simulink model "eulerEq"  (R2023b)
settings: Solver=ode4  StartTime=0.0  StopTime=30000  FixedStep=0.01  RelTol=1e-3
values from neighbouring files (symbols this model uses):
  date = [2023, 1, 21, 13, 52, 0]    [main.m]    (also in main_nonLin.m)
  euler0 = [0; 0; 0]    [main.m]    (also in main_nonLin.m)
  w0 = h0./sat.I'    [main.m]    (also in main_nonLin.m)
undefined symbols (not defined in the file or in its folder): airDensity, astroConstants, control, DiscIntNeverNeededParam, ea0, earth, gyroscope, magneticConstants, magnetorquer, magSensor, orbit, physicsConstants, rw, sat, sunSensor
libraries: simulink x21, matrix_library x7, sharedtransform x5, dspindex x5, sharedutil x4, vrlib x3, dspfactors x1, simulink_extras x1
(part 2 of 2)

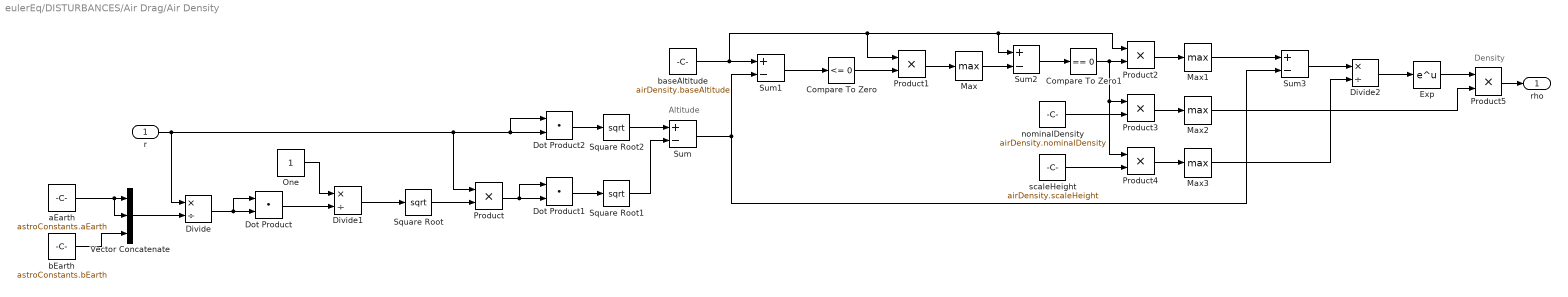
== system eulerEq/DISTURBANCES/Air Drag/Air Density ==
  note: Density
  note: Altitude
  r : Inport
  Compare To Zero : simulink/Logic and Bit Operations/Compare To Zero  relop=<=  OutDataTypeStr=boolean
  Compare To Zero1 : simulink/Logic and Bit Operations/Compare To Zero  relop===  OutDataTypeStr=boolean
  Divide : Product  Inputs=*/
  Divide1 : Product  Inputs=*/
  Divide2 : Product  Inputs=*/
  Dot Product : DotProduct  OutDataTypeStr=Inherit: Inherit via internal rule
  Dot Product1 : DotProduct  OutDataTypeStr=Inherit: Inherit via internal rule
  Dot Product2 : DotProduct  OutDataTypeStr=Inherit: Inherit via internal rule
  Exp : Math
  Max{,1..3} (4 alike) : MinMax  Function=max
  One : Constant  OutDataTypeStr=Inherit: Inherit via back propagation
  Product{,1..5} (6 alike) : Product
  Square Root : Sqrt
  Square Root1 : Sqrt
  Square Root2 : Sqrt
  Sum{,1..3} (4 alike) : Sum  Inputs=+-
  Vector Concatenate : Concatenate  NumInputs=3
  aEarth : Constant  Value=astroConstants.aEarth
  bEarth : Constant  Value=astroConstants.bEarth
  baseAltitude : Constant  Value=airDensity.baseAltitude
  nominalDensity : Constant  Value=airDensity.nominalDensity
  scaleHeight : Constant  Value=airDensity.scaleHeight
  rho : Outport
  wires:
  Product4/1 -> Max3/1
  Product/1 -> Dot Product1/1, Dot Product1/2
  Sum/1 -> Sum1/2, Sum3/2
  Max2/1 -> Product5/2
  Dot Product1/1 -> Square Root1/1
  Divide2/1 -> Exp/1
  Exp/1 -> Product5/1
  aEarth/1 -> Vector Concatenate/2, Vector Concatenate/1
  Product3/1 -> Max2/1
  Divide/1 -> Dot Product/1, Dot Product/2
  baseAltitude/1 -> Sum1/1, Product1/1, Sum2/1, Product2/1
  Max1/1 -> Sum3/1
  Dot Product/1 -> Divide1/2
  Max3/1 -> Divide2/2
  Compare To Zero1/1 -> Product2/2, Product4/1, Product3/1
  scaleHeight/1 -> Product4/2
  Dot Product2/1 -> Square Root2/1
  nominalDensity/1 -> Product3/2
  Sum1/1 -> Compare To Zero/1
  Square Root1/1 -> Sum/2
  Sum2/1 -> Compare To Zero1/1
  Sum3/1 -> Divide2/1
  Compare To Zero/1 -> Product1/2
  Product1/1 -> Max/1
  Product5/1 -> rho/1
  Max/1 -> Sum2/2
  bEarth/1 -> Vector Concatenate/3
  One/1 -> Divide1/1
  Divide1/1 -> Square Root/1
  Vector Concatenate/1 -> Divide/2
  Square Root2/1 -> Sum/1
  Square Root/1 -> Product/2
  Product2/1 -> Max1/1
  r/1 -> Divide/1, Dot Product2/1, Dot Product2/2, Product/1

== system eulerEq/DISTURBANCES/Air Drag/Matrix Cross Product ==
  a : Inport
  b : Inport  Port=2
  Add3 : Sum  Inputs=+-
  Add4 : Sum  Inputs=+-
  Add5 : Sum  Inputs=+-
  Matrix Concatenate2 : Concatenate  NumInputs=3  Mode=Multidimensional array
  Multiport Selector : dspindex/Multiport Selector  rowsOrCols=Rows  idxCellArray={1,2,3}  idxErrMode=Clip Index
  Multiport Selector1 : dspindex/Multiport Selector  rowsOrCols=Rows  idxCellArray={1,2,3}  idxErrMode=Clip Index
  Product{,1..2,11..13} (6 alike) : Product
  c : Outport
  wires:
  Product1/1 -> Add3/2
  Add4/1 -> Matrix Concatenate2/2
  Product11/1 -> Add4/2
  Multiport Selector/2 -> Product12/1, Product/1
  Product2/1 -> Add4/1
  Multiport Selector/1 -> Product11/1, Product13/1
  a/1 -> Multiport Selector/1
  Matrix Concatenate2/1 -> c/1
  b/1 -> Multiport Selector1/1
  Product12/1 -> Add5/2
  Multiport Selector1/3 -> Product11/2, Product/2
  Multiport Selector/3 -> Product1/1, Product2/1
  Multiport Selector1/1 -> Product12/2, Product2/2
  Multiport Selector1/2 -> Product1/2, Product13/2
  Add5/1 -> Matrix Concatenate2/3
  Product13/1 -> Add5/1
  Product/1 -> Add3/1
  Add3/1 -> Matrix Concatenate2/1

== system eulerEq/DISTURBANCES/Air Drag/Normalize ==
  V : Inport
  Divide3 : Product  Inputs=*/
  Dot Product3 : DotProduct  OutDataTypeStr=Inherit: Inherit via internal rule
  Square Root3 : Sqrt
  Vnorm : Outport
  wires:
  Square Root3/1 -> Divide3/2
  V/1 -> Divide3/1, Dot Product3/2, Dot Product3/1
  Dot Product3/1 -> Square Root3/1
  Divide3/1 -> Vnorm/1

== system eulerEq/DISTURBANCES/Gravity Gradient/Normalize2 ==
  r : Inport
  Dot Product : DotProduct  OutDataTypeStr=Inherit: Inherit via internal rule
  Product : Product  Inputs=*/
  Sqrt : Sqrt
  Out : Outport
  wires:
  Dot Product/1 -> Sqrt/1
  r/1 -> Dot Product/2, Dot Product/1, Product/1
  Sqrt/1 -> Product/2
  Product/1 -> Out/1

== system eulerEq/DISTURBANCES/SRP/Matrix Cross Product ==
  a : Inport
  b : Inport  Port=2
  Add3 : Sum  Inputs=+-
  Add4 : Sum  Inputs=+-
  Add5 : Sum  Inputs=+-
  Matrix Concatenate2 : Concatenate  NumInputs=3  Mode=Multidimensional array
  Multiport Selector : dspindex/Multiport Selector  rowsOrCols=Rows  idxCellArray={1,2,3}  idxErrMode=Clip Index
  Multiport Selector1 : dspindex/Multiport Selector  rowsOrCols=Rows  idxCellArray={1,2,3}  idxErrMode=Clip Index
  Product{,1..2,11..13} (6 alike) : Product
  c : Outport
  wires:
  Product1/1 -> Add3/2
  Add4/1 -> Matrix Concatenate2/2
  Product11/1 -> Add4/2
  Multiport Selector/2 -> Product12/1, Product/1
  Product2/1 -> Add4/1
  Multiport Selector/1 -> Product11/1, Product13/1
  a/1 -> Multiport Selector/1
  Matrix Concatenate2/1 -> c/1
  b/1 -> Multiport Selector1/1
  Product12/1 -> Add5/2
  Multiport Selector1/3 -> Product11/2, Product/2
  Multiport Selector/3 -> Product1/1, Product2/1
  Multiport Selector1/1 -> Product12/2, Product2/2
  Multiport Selector1/2 -> Product1/2, Product13/2
  Add5/1 -> Matrix Concatenate2/3
  Product13/1 -> Add5/1
  Product/1 -> Add3/1
  Add3/1 -> Matrix Concatenate2/1

== system eulerEq/KINEMATICS/312 Subsystem/Kinematics Euler Angles 312 ==
  Euler Angles : Inport
  Angular Velocity : Inport  Port=2
  Add : Sum  Inputs=+-
  Add1 : Sum
  Add2 : Sum  Inputs=+-
  Cos1 : Trigonometry  Operator=cos
  Cos2 : Trigonometry  Operator=cos
  Demux : Demux  Outputs=3
  Demux1 : Demux  Outputs=3
  Divide1 : Product  Inputs=*/
  Mux : Mux  Inputs=3
  Product7 : Product
  Sin1 : Trigonometry
  Sin2 : Trigonometry
  Terminator : Terminator
  Wu*cos(psi) : Product
  Wu*sin(psi) : Product
  Ww*cos(psi) : Product
  Ww*sin(psi) : Product
  Euler Angles Dot : Outport
  wires:
  Add/1 -> Divide1/1
  Demux/1 -> Wu*cos(psi)/1, Wu*sin(psi)/2  "Wu"
  Product7/1 -> Add2/2
  Wu*sin(psi)/1 -> Add/2
  Sin2/1 -> Wu*sin(psi)/1, Ww*sin(psi)/2
  Demux1/3 -> Cos2/1, Sin2/1  "psi"
  Demux1/1 -> Terminator/1  "phi"
  Euler Angles/1 -> Demux1/1
  Sin1/1 -> Product7/2
  Mux/1 -> Euler Angles Dot/1
  Divide1/1 -> Product7/1, Mux/1  "phi dot"
  Demux/2 -> Add2/1  "Wv"
  Demux/3 -> Ww*sin(psi)/1, Ww*cos(psi)/2  "Ww"
  Ww*sin(psi)/1 -> Add1/2
  Cos2/1 -> Ww*cos(psi)/1, Wu*cos(psi)/2
  Add1/1 -> Mux/2  "theta dot"
  Cos1/1 -> Divide1/2
  Demux1/2 -> Sin1/1, Cos1/1  "theta"
  Wu*cos(psi)/1 -> Add1/1
  Angular Velocity/1 -> Demux/1
  Ww*cos(psi)/1 -> Add/1
  Add2/1 -> Mux/3  "psi dot"

== system eulerEq/KINEMATICS/312 Subsystem/rotmToEul 312 ==
  In1 : Inport
  Create 3x3 Matrix : sharedutil/Create 3x3 Matrix  aMode=aMode
  Fcn11 : Fcn  Expr=u(6)*u(4) - u(2)*u(3)*u(1)
  Fcn12 : Fcn  Expr=u(6)*u(1) + u(2)*u(3)*u(4)
  Fcn13 : Fcn  Expr=-u(3)*u(5)
  Fcn21 : Fcn  Expr=-u(5)*u(1)
  Fcn22 : Fcn  Expr=u(5)*u(4)
  Fcn23 : Fcn  Expr=u(2)
  Fcn31 : Fcn  Expr=u(3)*u(4) + u(2)*u(6)*u(1)
  Fcn32 : Fcn  Expr=u(3)*u(1) - u(2)*u(6)*u(4)
  Fcn33 : Fcn  Expr=u(5)*u(6)
  Mux : Mux  Inputs=2
  sincos : Trigonometry  Operator=sincos
  Out1 : Outport
  wires:
  sincos/2 -> Mux/2
  Fcn22/1 -> Create 3x3 Matrix/5
  Fcn13/1 -> Create 3x3 Matrix/3
  Fcn31/1 -> Create 3x3 Matrix/7
  Mux/1 -> Fcn11/1, Fcn12/1, Fcn13/1, Fcn21/1, Fcn32/1, Fcn33/1, Fcn31/1, Fcn23/1, Fcn22/1
  Fcn21/1 -> Create 3x3 Matrix/4
  Fcn12/1 -> Create 3x3 Matrix/2
  Fcn32/1 -> Create 3x3 Matrix/8
  Fcn33/1 -> Create 3x3 Matrix/9
  Fcn11/1 -> Create 3x3 Matrix/1
  Fcn23/1 -> Create 3x3 Matrix/6
  sincos/1 -> Mux/1
  Create 3x3 Matrix/1 -> Out1/1
  In1/1 -> sincos/1

== system eulerEq/KINEMATICS/313 Subsystem/Kinematics Euler Angles 313 ==
  Angular Velocity : Inport
  Euler Angles : Inport  Port=2
  Add : Sum
  Add1 : Sum  Inputs=+-
  Add2 : Sum  Inputs=+-
  Cos1 : Trigonometry  Operator=cos
  Cos2 : Trigonometry  Operator=cos
  Demux : Demux  Outputs=3
  Demux1 : Demux  Outputs=3
  Divide1 : Product  Inputs=*/
  Mux : Mux  Inputs=3
  Product7 : Product
  Sin1 : Trigonometry
  Sin2 : Trigonometry
  Terminator : Terminator
  Wu*cos(psi) : Product
  Wu*sin(psi) : Product
  Wv*cos(psi) : Product
  Wv*sin(psi) : Product
  Euler Angles Dot : Outport
  wires:
  Add/1 -> Divide1/1
  Demux/1 -> Wu*cos(psi)/1, Wu*sin(psi)/2  "Wu"
  Wv*cos(psi)/1 -> Add/2
  Sin2/1 -> Wv*sin(psi)/2, Wu*sin(psi)/1
  Demux1/3 -> Cos2/1, Sin2/1  "psi"
  Demux1/1 -> Terminator/1  "phi"
  Euler Angles/1 -> Demux1/1
  Sin1/1 -> Divide1/2
  Mux/1 -> Euler Angles Dot/1
  Divide1/1 -> Product7/2, Mux/1  "phi dot"
  Demux/2 -> Wv*sin(psi)/1, Wv*cos(psi)/2  "Wv"
  Demux/3 -> Add2/1  "Ww"
  Wv*sin(psi)/1 -> Add1/2
  Cos2/1 -> Wu*cos(psi)/2, Wv*cos(psi)/1
  Add1/1 -> Mux/2  "theta dot"
  Demux1/2 -> Sin1/1, Cos1/1  "theta"
  Wu*cos(psi)/1 -> Add1/1
  Angular Velocity/1 -> Demux/1
  Wu*sin(psi)/1 -> Add/1
  Add2/1 -> Mux/3  "psi dot"
  Product7/1 -> Add2/2
  Cos1/1 -> Product7/1

== system eulerEq/KINEMATICS/313 Subsystem/rotmToEul 313 ==
  In1 : Inport
  Create 3x3 Matrix : sharedutil/Create 3x3 Matrix  aMode=aMode
  Fcn11 : Fcn  Expr=-u(1)*u(5)*u(3) + u(4)*u(6)
  Fcn12 : Fcn  Expr=u(4)*u(5)*u(3) + u(1)*u(6)
  Fcn13 : Fcn  Expr=u(2)*u(3)
  Fcn21 : Fcn  Expr=-u(1)*u(6)*u(5) - u(4)*u(3)
  Fcn22 : Fcn  Expr=u(4)*u(6)*u(5) - u(1)*u(3)
  Fcn23 : Fcn  Expr=u(2)*u(6)
  Fcn31 : Fcn  Expr=u(1)*u(2)
  Fcn32 : Fcn  Expr=-u(4)*u(2)
  Fcn33 : Fcn  Expr=u(5)
  Mux : Mux  Inputs=2
  sincos : Trigonometry  Operator=sincos
  Out1 : Outport
  wires:
  sincos/1 -> Mux/1
  Fcn22/1 -> Create 3x3 Matrix/5
  sincos/2 -> Mux/2
  Fcn13/1 -> Create 3x3 Matrix/3
  Fcn23/1 -> Create 3x3 Matrix/6
  Fcn11/1 -> Create 3x3 Matrix/1
  Mux/1 -> Fcn11/1, Fcn12/1, Fcn13/1, Fcn21/1, Fcn32/1, Fcn33/1, Fcn31/1, Fcn23/1, Fcn22/1
  Fcn12/1 -> Create 3x3 Matrix/2
  Fcn31/1 -> Create 3x3 Matrix/7
  Create 3x3 Matrix/1 -> Out1/1
  Fcn32/1 -> Create 3x3 Matrix/8
  Fcn21/1 -> Create 3x3 Matrix/4
  Fcn33/1 -> Create 3x3 Matrix/9
  In1/1 -> sincos/1

== system eulerEq/KINEMATICS/Initial Conditions/rotmToEa 312 ==
  A : Inport
  Enable : EnablePort
  Direction Cosine Matrix to Rotation Angles : sharedtransform/Direction Cosine Matrix to Rotation Angles  rotationOrder=ZXY  aMode=aMode  action=None  tolerance=eps(2)
      settings: LibrarySourceBlock=|
      | aerolibtransform2/Direction Cosine Matrix
      | to Rotation Angles
  ea : Outport  InitialOutput=zeros(1,3)
  wires:
  A/1 -> Direction Cosine Matrix to Rotation Angles/1
  Direction Cosine Matrix to Rotation Angles/1 -> ea/1

== system eulerEq/KINEMATICS/Initial Conditions/rotmToEa 313 ==
  A : Inport
  Enable : EnablePort
  Direction Cosine Matrix to Rotation Angles : sharedtransform/Direction Cosine Matrix to Rotation Angles  rotationOrder=ZXZ  aMode=aMode  action=None  tolerance=eps(2)
      settings: LibrarySourceBlock=|
      | aerolibtransform2/Direction Cosine Matrix
      | to Rotation Angles
  ea : Outport  InitialOutput=zeros(1,3)
  wires:
  Direction Cosine Matrix to Rotation Angles/1 -> ea/1
  A/1 -> Direction Cosine Matrix to Rotation Angles/1

== matlab function eulerEq/ATTITUDE DETERMINATION/Magnetic Field/MATLAB Function ==
  data: r input; B output; T input; date input; igrfSg input; igrfSh input
function B = fcn(r, T, date, igrfSg, igrfSh)

B = [0;0;0];

days = date2mjd2000(date) + T/86400;

[rNorm, lat, lon] = carToGCS(r, T);
[Br,Bt,Bp] = magnet(rNorm,lat,lon,days,igrfSg,igrfSh);

LST = calculateLST(date, lon);

[Bx,By,Bz] = msph2inert(Br,Bt,Bp,LST,lat);
B = [Bx; By; Bz];
end
